simulink model "Simulation_of_sysGit"  (R2020b)
settings: Solver=VariableStepAuto  StartTime=0.0  StopTime=10.0  RelTol=1e-3
values from neighbouring files (symbols this model uses):
  S = pi*a^2    (= 1.96349540849e-05)    [bodeplot.m]
  S_FV = 20*log10(abs(S_FV))    [bodeplot.m]
  w = linspace(1,2.5*pi*f,10000)    [bodeplot.m]
settings Model: Creator=hoejb  LastModifiedBy=hoejb

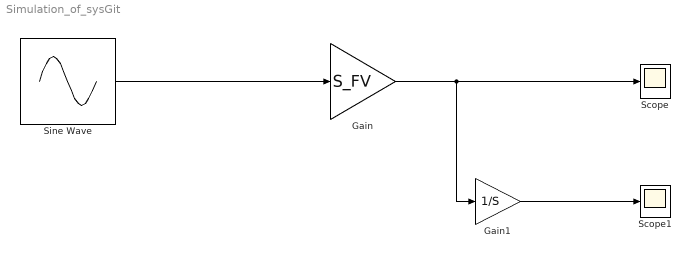
== system Simulation_of_sysGit ==
  Gain : Gain  Gain=S_FV
  Gain1 : Gain  Gain=1/S
  Scope : Scope
  Scope1 : Scope
  Sine Wave : Sin  Amplitude=300  Frequency=w  SampleTime=0
  wires:
  Gain/1 -> Gain1/1, Scope/1
  Gain1/1 -> Scope1/1
  Sine Wave/1 -> Gain/1
